simulink model "nms_3Dmodel_nonlin"  (R2019a)
settings: Solver=ode15s  StartTime=0.0  StopTime=10  FixedStep=1e-3  RelTol=1e-3  AbsTol=1e-4  EnableMultiTasking=on
InitFcn:
  | runScripts;
undefined symbols (not defined in the file or in its folder): ankle_height, c, c_jointstop, CtrlPar_FP, CtrlPar_FP_R, CtrlPar_LL, CtrlPar_St, CtrlPar_St_R, CtrlPar_Sw, CtrlPar_Sw_R, CtrlPar_theta0, CtrlPar_Tr, CtrlPar_Tr_R, D12_F, D12_S, D12_T, D12z_T, D13_F, D1G_F, D1G_HAT, D1G_S, D1G_T, D1Gy_F, d_fBall, d_fHeel, DeltaThRef, dt, eref, FmaxBFSH, FmaxGAS, FmaxGLU, FmaxHAB, FmaxHAD, FmaxHAM, FmaxHFL, FmaxRF, FmaxSOL, FmaxTA, FmaxVAS, In_F, In_HAT, In_S, In_T, init_a_tgt, init_a_tgtR, Inx_F, Inx_HAT, Inx_S, Inx_T, Iny_F, Iny_HAT, Iny_S, Iny_T, K, k_gn, k_gt, k_pressure, leg_l, LongDelay, LongLoopDelay ... (+139)
libraries: mblibv1 x89, simulink x44, simulink_extras x38
(part 11 of 13)

== system nms_3Dmodel_nonlin/Muscle Actuation Layer/R RF/PE force-length relation ==
  note: Parallel Elasticity PE
  lce [lopt] : Inport
  Constant3 : Constant
  Math Function2 : Math  Operator=square  SaturateOnIntegerOverflow=on
  Mux : Mux  Inputs=2
  Sum1 : Sum  Inputs=|+-  SaturateOnIntegerOverflow=on  InputSameDT=on  OutDataTypeStr=Inherit: Same as first input
  force above slack length : Fcn  Expr=u(2) * (u(1)>1)
  reference strain [lopt] : Constant  Value=w
  relative strain : Product  Inputs=*/
  fpe [Fmax] : Outport
  wires:
  Mux/1 -> force above slack length/1
  lce [lopt]/1 -> Mux/1, Sum1/1
  Constant3/1 -> Sum1/2
  Sum1/1 -> relative strain/1
  reference strain [lopt]/1 -> relative strain/2
  relative strain/1 -> Math Function2/1
  Math Function2/1 -> Mux/2
  force above slack length/1 -> fpe [Fmax]/1

== system nms_3Dmodel_nonlin/Muscle Actuation Layer/R RF/SE force-length relation ==
  note: SE Force-Length Relationship
  lse [lslack] : Inport
  Constant1 : Constant
  Math Function : Math  Operator=square  SaturateOnIntegerOverflow=on
  Mux : Mux  Inputs=2
  Sum4 : Sum  Inputs=|+-  SaturateOnIntegerOverflow=on  InputSameDT=on  OutDataTypeStr=Inherit: Same as first input
  force above slack length : Fcn  Expr=u(2)*(u(1)>1)
  reference strain [lslack] : Constant  Value=eref
  relative strain : Product  Inputs=*/
  fse [Fmax] : Outport
  wires:
  Mux/1 -> force above slack length/1
  force above slack length/1 -> fse [Fmax]/1
  Math Function/1 -> Mux/2
  lse [lslack]/1 -> Mux/1, Sum4/1
  relative strain/1 -> Math Function/1
  reference strain [lslack]/1 -> relative strain/2
  Sum4/1 -> relative strain/1
  Constant1/1 -> Sum4/2

== system nms_3Dmodel_nonlin/Muscle Actuation Layer/R SOL/BE force-length relation ==
  note: Buffer Elasticity BE
  lce [lopt] : Inport
  Constant1 : Constant  Value=1-w
  Math Function : Math  Operator=square  SaturateOnIntegerOverflow=on
  Mux1 : Mux  Inputs=2
  Sum4 : Sum  Inputs=|+-  SaturateOnIntegerOverflow=on  InputSameDT=on  OutDataTypeStr=Inherit: Same as first input
  force above slack length : Fcn  Expr=u(2)*(u(1)<0)
  reference strain [lslack] : Constant  Value=w/2
  relative strain : Product  Inputs=*/
  fbe [Fmax] : Outport
  wires:
  lce [lopt]/1 -> Sum4/1
  Mux1/1 -> force above slack length/1
  force above slack length/1 -> fbe [Fmax]/1
  Math Function/1 -> Mux1/2
  relative strain/1 -> Math Function/1
  reference strain [lslack]/1 -> relative strain/2
  Sum4/1 -> relative strain/1, Mux1/1
  Constant1/1 -> Sum4/2

== system nms_3Dmodel_nonlin/Muscle Actuation Layer/R SOL/CE force-length relation ==
  note: CE Force-Length Relationship
  lce [lopt] : Inport
  Abs : Abs
  Constant1 : Constant
  Constant2 : Constant  Value=3
  Gain : Gain  Gain=log(c)
  Math Function : Math  SaturateOnIntegerOverflow=on
  Math Function1 : Math  Operator=pow  SaturateOnIntegerOverflow=on
  Sum4 : Sum  Inputs=|+-  SaturateOnIntegerOverflow=on  InputSameDT=on  OutDataTypeStr=Inherit: Same as first input
  normalized position : Product  Inputs=*/
  relative width : Constant  Value=w
  fce [Fmax] : Outport
  wires:
  lce [lopt]/1 -> Sum4/1
  relative width/1 -> normalized position/2
  Constant1/1 -> Sum4/2
  Sum4/1 -> Abs/1
  Abs/1 -> normalized position/1
  normalized position/1 -> Math Function1/1
  Constant2/1 -> Math Function1/2
  Math Function1/1 -> Gain/1
  Gain/1 -> Math Function/1
  Math Function/1 -> fce [Fmax]/1

== system nms_3Dmodel_nonlin/Muscle Actuation Layer/R SOL/CE inverse force-velocity relation ==
  note: CE Inverse Force-Velocity Relationship
  Fv[Fmax] : Inport
  1 : Product  Inputs=/*
  Constant{1,3..4,8} (4 alike) : Constant
  Constant2 : Constant  Value=N
  Constant5 : Constant  Value=N
  Curvature : Gain  Gain=K  SaturateOnIntegerOverflow=on  OutDataTypeStr=Inherit: Same as input  ParamDataTypeStr=Inherit: Same as input
  Curvature1 : Gain  Gain=7.56*K  SaturateOnIntegerOverflow=on  OutDataTypeStr=Inherit: Same as input  ParamDataTypeStr=Inherit: Same as input
  Mux : Mux  Inputs=2
  Mux1 : Mux  Inputs=3
  Mux2 : Mux  Inputs=3
  Slope : Gain  Gain=1e-2  SaturateOnIntegerOverflow=on  OutDataTypeStr=Inherit: Same as input  ParamDataTypeStr=Inherit: Same as input
  Sum1 : Sum  Inputs=|++  SaturateOnIntegerOverflow=on  InputSameDT=on  OutDataTypeStr=Inherit: Same as first input
  Sum2 : Sum  SaturateOnIntegerOverflow=on  InputSameDT=on  OutDataTypeStr=Inherit: Same as first input
  Sum3 : Sum  Inputs=++|  SaturateOnIntegerOverflow=on  InputSameDT=on  OutDataTypeStr=Inherit: Same as first input
  Sum4 : Sum  Inputs=|+-  SaturateOnIntegerOverflow=on  InputSameDT=on  OutDataTypeStr=Inherit: Same as first input
  Sum5 : Sum  Inputs=|-+  SaturateOnIntegerOverflow=on  InputSameDT=on  OutDataTypeStr=Inherit: Same as first input
  Sum6 : Sum  Inputs=-+|  SaturateOnIntegerOverflow=on  InputSameDT=on  OutDataTypeStr=Inherit: Same as first input
  Sum7 : Sum  Inputs=|++  SaturateOnIntegerOverflow=on  InputSameDT=on  OutDataTypeStr=Inherit: Same as first input
  Sum8 : Sum  Inputs=+-|  SaturateOnIntegerOverflow=on  InputSameDT=on  OutDataTypeStr=Inherit: Same as first input
  Sum9 : Sum  SaturateOnIntegerOverflow=on  InputSameDT=on  OutDataTypeStr=Inherit: Same as first input
  concentric branch : Fcn  Expr=u(1) * (u(2)<=1)
  excentric branch : Fcn  Expr=u(2) * (u(1)>1)*(u(1)<=u(3))
  excentric overshoot : Fcn  Expr=u(3) * (u(2)>u(1))
  v_concentric : Product  Inputs=*/
  v_excentric <N : Product  Inputs=*/
  v[vmax] : Outport
  wires:
  Curvature/1 -> Sum3/2
  Constant1/1 -> Sum4/2, Sum3/1
  Sum4/1 -> v_concentric/1
  Sum3/1 -> v_concentric/2
  1/1 -> Sum7/1, Curvature1/1
  Constant4/1 -> Sum7/2, Sum8/1
  Curvature1/1 -> Sum8/2
  Sum8/1 -> v_excentric <N/2
  Sum7/1 -> v_excentric <N/1
  v_concentric/1 -> Mux/1
  Fv[Fmax]/1 -> Sum4/1, Curvature/1, Sum6/2, Mux/2, Mux1/1, Mux2/2
  Sum9/1 -> v[vmax]/1
  Sum2/1 -> Sum9/2
  excentric overshoot/1 -> Sum2/2
  Slope/1 -> Sum1/1
  Constant8/1 -> Sum1/2
  Sum6/1 -> 1/2, Slope/1
  Constant2/1 -> Sum6/1, Sum5/2
  Sum5/1 -> 1/1
  Constant3/1 -> Sum5/1
  Mux/1 -> concentric branch/1
  Mux1/1 -> excentric branch/1
  v_excentric <N/1 -> Mux1/2
  Mux2/1 -> excentric overshoot/1
  concentric branch/1 -> Sum9/1
  excentric branch/1 -> Sum2/1
  Constant5/1 -> Mux1/3, Mux2/1
  Sum1/1 -> Mux2/3

== system nms_3Dmodel_nonlin/Muscle Actuation Layer/R SOL/PE force-length relation ==
  note: Parallel Elasticity PE
  lce [lopt] : Inport
  Constant3 : Constant
  Math Function2 : Math  Operator=square  SaturateOnIntegerOverflow=on
  Mux : Mux  Inputs=2
  Sum1 : Sum  Inputs=|+-  SaturateOnIntegerOverflow=on  InputSameDT=on  OutDataTypeStr=Inherit: Same as first input
  force above slack length : Fcn  Expr=u(2) * (u(1)>1)
  reference strain [lopt] : Constant  Value=w
  relative strain : Product  Inputs=*/
  fpe [Fmax] : Outport
  wires:
  Mux/1 -> force above slack length/1
  lce [lopt]/1 -> Mux/1, Sum1/1
  Constant3/1 -> Sum1/2
  Sum1/1 -> relative strain/1
  reference strain [lopt]/1 -> relative strain/2
  relative strain/1 -> Math Function2/1
  Math Function2/1 -> Mux/2
  force above slack length/1 -> fpe [Fmax]/1

== system nms_3Dmodel_nonlin/Muscle Actuation Layer/R SOL/SE force-length relation ==
  note: SE Force-Length Relationship
  lse [lslack] : Inport
  Constant1 : Constant
  Math Function : Math  Operator=square  SaturateOnIntegerOverflow=on
  Mux : Mux  Inputs=2
  Sum4 : Sum  Inputs=|+-  SaturateOnIntegerOverflow=on  InputSameDT=on  OutDataTypeStr=Inherit: Same as first input
  force above slack length : Fcn  Expr=u(2)*(u(1)>1)
  reference strain [lslack] : Constant  Value=eref
  relative strain : Product  Inputs=*/
  fse [Fmax] : Outport
  wires:
  Mux/1 -> force above slack length/1
  force above slack length/1 -> fse [Fmax]/1
  Math Function/1 -> Mux/2
  lse [lslack]/1 -> Mux/1, Sum4/1
  relative strain/1 -> Math Function/1
  reference strain [lslack]/1 -> relative strain/2
  Sum4/1 -> relative strain/1
  Constant1/1 -> Sum4/2

== system nms_3Dmodel_nonlin/Muscle Actuation Layer/R TA/BE force-length relation ==
  note: Buffer Elasticity BE
  lce [lopt] : Inport
  Constant1 : Constant  Value=1-w
  Math Function : Math  Operator=square  SaturateOnIntegerOverflow=on
  Mux1 : Mux  Inputs=2
  Sum4 : Sum  Inputs=|+-  SaturateOnIntegerOverflow=on  InputSameDT=on  OutDataTypeStr=Inherit: Same as first input
  force above slack length : Fcn  Expr=u(2)*(u(1)<0)
  reference strain [lslack] : Constant  Value=w/2
  relative strain : Product  Inputs=*/
  fbe [Fmax] : Outport
  wires:
  lce [lopt]/1 -> Sum4/1
  Mux1/1 -> force above slack length/1
  force above slack length/1 -> fbe [Fmax]/1
  Math Function/1 -> Mux1/2
  relative strain/1 -> Math Function/1
  reference strain [lslack]/1 -> relative strain/2
  Sum4/1 -> relative strain/1, Mux1/1
  Constant1/1 -> Sum4/2

== system nms_3Dmodel_nonlin/Muscle Actuation Layer/R TA/CE force-length relation ==
  note: CE Force-Length Relationship
  lce [lopt] : Inport
  Abs : Abs
  Constant1 : Constant
  Constant2 : Constant  Value=3
  Gain : Gain  Gain=log(c)
  Math Function : Math  SaturateOnIntegerOverflow=on
  Math Function1 : Math  Operator=pow  SaturateOnIntegerOverflow=on
  Sum4 : Sum  Inputs=|+-  SaturateOnIntegerOverflow=on  InputSameDT=on  OutDataTypeStr=Inherit: Same as first input
  normalized position : Product  Inputs=*/
  relative width : Constant  Value=w
  fce [Fmax] : Outport
  wires:
  Math Function/1 -> fce [Fmax]/1
  Gain/1 -> Math Function/1
  Math Function1/1 -> Gain/1
  Constant2/1 -> Math Function1/2
  normalized position/1 -> Math Function1/1
  Abs/1 -> normalized position/1
  Sum4/1 -> Abs/1
  Constant1/1 -> Sum4/2
  relative width/1 -> normalized position/2
  lce [lopt]/1 -> Sum4/1

== system nms_3Dmodel_nonlin/Muscle Actuation Layer/R TA/CE inverse force-velocity relation ==
  note: CE Inverse Force-Velocity Relationship
  Fv[Fmax] : Inport
  1 : Product  Inputs=/*
  Constant{1,3..4,8} (4 alike) : Constant
  Constant2 : Constant  Value=N
  Constant5 : Constant  Value=N
  Curvature : Gain  Gain=K  SaturateOnIntegerOverflow=on  OutDataTypeStr=Inherit: Same as input  ParamDataTypeStr=Inherit: Same as input
  Curvature1 : Gain  Gain=7.56*K  SaturateOnIntegerOverflow=on  OutDataTypeStr=Inherit: Same as input  ParamDataTypeStr=Inherit: Same as input
  Mux : Mux  Inputs=2
  Mux1 : Mux  Inputs=3
  Mux2 : Mux  Inputs=3
  Slope : Gain  Gain=1e-2  SaturateOnIntegerOverflow=on  OutDataTypeStr=Inherit: Same as input  ParamDataTypeStr=Inherit: Same as input
  Sum1 : Sum  Inputs=|++  SaturateOnIntegerOverflow=on  InputSameDT=on  OutDataTypeStr=Inherit: Same as first input
  Sum2 : Sum  SaturateOnIntegerOverflow=on  InputSameDT=on  OutDataTypeStr=Inherit: Same as first input
  Sum3 : Sum  Inputs=++|  SaturateOnIntegerOverflow=on  InputSameDT=on  OutDataTypeStr=Inherit: Same as first input
  Sum4 : Sum  Inputs=|+-  SaturateOnIntegerOverflow=on  InputSameDT=on  OutDataTypeStr=Inherit: Same as first input
  Sum5 : Sum  Inputs=|-+  SaturateOnIntegerOverflow=on  InputSameDT=on  OutDataTypeStr=Inherit: Same as first input
  Sum6 : Sum  Inputs=-+|  SaturateOnIntegerOverflow=on  InputSameDT=on  OutDataTypeStr=Inherit: Same as first input
  Sum7 : Sum  Inputs=|++  SaturateOnIntegerOverflow=on  InputSameDT=on  OutDataTypeStr=Inherit: Same as first input
  Sum8 : Sum  Inputs=+-|  SaturateOnIntegerOverflow=on  InputSameDT=on  OutDataTypeStr=Inherit: Same as first input
  Sum9 : Sum  SaturateOnIntegerOverflow=on  InputSameDT=on  OutDataTypeStr=Inherit: Same as first input
  concentric branch : Fcn  Expr=u(1) * (u(2)<=1)
  excentric branch : Fcn  Expr=u(2) * (u(1)>1)*(u(1)<=u(3))
  excentric overshoot : Fcn  Expr=u(3) * (u(2)>u(1))
  v_concentric : Product  Inputs=*/
  v_excentric <N : Product  Inputs=*/
  v[vmax] : Outport
  wires:
  Sum1/1 -> Mux2/3
  Constant5/1 -> Mux2/1, Mux1/3
  excentric branch/1 -> Sum2/1
  concentric branch/1 -> Sum9/1
  Mux2/1 -> excentric overshoot/1
  v_excentric <N/1 -> Mux1/2
  Mux1/1 -> excentric branch/1
  Mux/1 -> concentric branch/1
  Constant3/1 -> Sum5/1
  Sum5/1 -> 1/1
  Constant2/1 -> Sum5/2, Sum6/1
  Sum6/1 -> Slope/1, 1/2
  Constant8/1 -> Sum1/2
  Slope/1 -> Sum1/1
  excentric overshoot/1 -> Sum2/2
  Sum2/1 -> Sum9/2
  Sum9/1 -> v[vmax]/1
  Fv[Fmax]/1 -> Mux2/2, Mux1/1, Mux/2, Sum6/2, Curvature/1, Sum4/1
  v_concentric/1 -> Mux/1
  Sum7/1 -> v_excentric <N/1
  Sum8/1 -> v_excentric <N/2
  Curvature1/1 -> Sum8/2
  Constant4/1 -> Sum8/1, Sum7/2
  1/1 -> Curvature1/1, Sum7/1
  Sum3/1 -> v_concentric/2
  Sum4/1 -> v_concentric/1
  Constant1/1 -> Sum3/1, Sum4/2
  Curvature/1 -> Sum3/2

== system nms_3Dmodel_nonlin/Muscle Actuation Layer/R TA/PE force-length relation ==
  note: Parallel Elasticity PE
  lce [lopt] : Inport
  Constant3 : Constant
  Math Function2 : Math  Operator=square  SaturateOnIntegerOverflow=on
  Mux : Mux  Inputs=2
  Sum1 : Sum  Inputs=|+-  SaturateOnIntegerOverflow=on  InputSameDT=on  OutDataTypeStr=Inherit: Same as first input
  force above slack length : Fcn  Expr=u(2) * (u(1)>1)
  reference strain [lopt] : Constant  Value=w
  relative strain : Product  Inputs=*/
  fpe [Fmax] : Outport
  wires:
  Mux/1 -> force above slack length/1
  lce [lopt]/1 -> Mux/1, Sum1/1
  Constant3/1 -> Sum1/2
  Sum1/1 -> relative strain/1
  reference strain [lopt]/1 -> relative strain/2
  relative strain/1 -> Math Function2/1
  Math Function2/1 -> Mux/2
  force above slack length/1 -> fpe [Fmax]/1

== system nms_3Dmodel_nonlin/Muscle Actuation Layer/R TA/SE force-length relation ==
  note: SE Force-Length Relationship
  lse [lslack] : Inport
  Constant1 : Constant
  Math Function : Math  Operator=square  SaturateOnIntegerOverflow=on
  Mux : Mux  Inputs=2
  Sum4 : Sum  Inputs=|+-  SaturateOnIntegerOverflow=on  InputSameDT=on  OutDataTypeStr=Inherit: Same as first input
  force above slack length : Fcn  Expr=u(2)*(u(1)>1)
  reference strain [lslack] : Constant  Value=eref
  relative strain : Product  Inputs=*/
  fse [Fmax] : Outport
  wires:
  Mux/1 -> force above slack length/1
  force above slack length/1 -> fse [Fmax]/1
  Math Function/1 -> Mux/2
  lse [lslack]/1 -> Mux/1, Sum4/1
  relative strain/1 -> Math Function/1
  reference strain [lslack]/1 -> relative strain/2
  Sum4/1 -> relative strain/1
  Constant1/1 -> Sum4/2

== system nms_3Dmodel_nonlin/Muscle Actuation Layer/R VAS/BE force-length relation ==
  note: Buffer Elasticity BE
  lce [lopt] : Inport
  Constant1 : Constant  Value=1-w
  Math Function : Math  Operator=square  SaturateOnIntegerOverflow=on
  Mux1 : Mux  Inputs=2
  Sum4 : Sum  Inputs=|+-  SaturateOnIntegerOverflow=on  InputSameDT=on  OutDataTypeStr=Inherit: Same as first input
  force above slack length : Fcn  Expr=u(2)*(u(1)<0)
  reference strain [lslack] : Constant  Value=w/2
  relative strain : Product  Inputs=*/
  fbe [Fmax] : Outport
  wires:
  lce [lopt]/1 -> Sum4/1
  Mux1/1 -> force above slack length/1
  force above slack length/1 -> fbe [Fmax]/1
  Math Function/1 -> Mux1/2
  relative strain/1 -> Math Function/1
  reference strain [lslack]/1 -> relative strain/2
  Sum4/1 -> relative strain/1, Mux1/1
  Constant1/1 -> Sum4/2

== system nms_3Dmodel_nonlin/Muscle Actuation Layer/R VAS/CE force-length relation ==
  note: CE Force-Length Relationship
  lce [lopt] : Inport
  Abs : Abs
  Constant1 : Constant
  Constant2 : Constant  Value=3
  Gain : Gain  Gain=log(c)
  Math Function : Math  SaturateOnIntegerOverflow=on
  Math Function1 : Math  Operator=pow  SaturateOnIntegerOverflow=on
  Sum4 : Sum  Inputs=|+-  SaturateOnIntegerOverflow=on  InputSameDT=on  OutDataTypeStr=Inherit: Same as first input
  normalized position : Product  Inputs=*/
  relative width : Constant  Value=w
  fce [Fmax] : Outport
  wires:
  lce [lopt]/1 -> Sum4/1
  relative width/1 -> normalized position/2
  Constant1/1 -> Sum4/2
  Sum4/1 -> Abs/1
  Abs/1 -> normalized position/1
  normalized position/1 -> Math Function1/1
  Constant2/1 -> Math Function1/2
  Math Function1/1 -> Gain/1
  Gain/1 -> Math Function/1
  Math Function/1 -> fce [Fmax]/1

== system nms_3Dmodel_nonlin/Muscle Actuation Layer/R VAS/CE inverse force-velocity relation ==
  note: CE Inverse Force-Velocity Relationship
  Fv[Fmax] : Inport
  1 : Product  Inputs=/*
  Constant{1,3..4,8} (4 alike) : Constant
  Constant2 : Constant  Value=N
  Constant5 : Constant  Value=N
  Curvature : Gain  Gain=K  SaturateOnIntegerOverflow=on  OutDataTypeStr=Inherit: Same as input  ParamDataTypeStr=Inherit: Same as input
  Curvature1 : Gain  Gain=7.56*K  SaturateOnIntegerOverflow=on  OutDataTypeStr=Inherit: Same as input  ParamDataTypeStr=Inherit: Same as input
  Mux : Mux  Inputs=2
  Mux1 : Mux  Inputs=3
  Mux2 : Mux  Inputs=3
  Slope : Gain  Gain=1e-2  SaturateOnIntegerOverflow=on  OutDataTypeStr=Inherit: Same as input  ParamDataTypeStr=Inherit: Same as input
  Sum1 : Sum  Inputs=|++  SaturateOnIntegerOverflow=on  InputSameDT=on  OutDataTypeStr=Inherit: Same as first input
  Sum2 : Sum  SaturateOnIntegerOverflow=on  InputSameDT=on  OutDataTypeStr=Inherit: Same as first input
  Sum3 : Sum  Inputs=++|  SaturateOnIntegerOverflow=on  InputSameDT=on  OutDataTypeStr=Inherit: Same as first input
  Sum4 : Sum  Inputs=|+-  SaturateOnIntegerOverflow=on  InputSameDT=on  OutDataTypeStr=Inherit: Same as first input
  Sum5 : Sum  Inputs=|-+  SaturateOnIntegerOverflow=on  InputSameDT=on  OutDataTypeStr=Inherit: Same as first input
  Sum6 : Sum  Inputs=-+|  SaturateOnIntegerOverflow=on  InputSameDT=on  OutDataTypeStr=Inherit: Same as first input
  Sum7 : Sum  Inputs=|++  SaturateOnIntegerOverflow=on  InputSameDT=on  OutDataTypeStr=Inherit: Same as first input
  Sum8 : Sum  Inputs=+-|  SaturateOnIntegerOverflow=on  InputSameDT=on  OutDataTypeStr=Inherit: Same as first input
  Sum9 : Sum  SaturateOnIntegerOverflow=on  InputSameDT=on  OutDataTypeStr=Inherit: Same as first input
  concentric branch : Fcn  Expr=u(1) * (u(2)<=1)
  excentric branch : Fcn  Expr=u(2) * (u(1)>1)*(u(1)<=u(3))
  excentric overshoot : Fcn  Expr=u(3) * (u(2)>u(1))
  v_concentric : Product  Inputs=*/
  v_excentric <N : Product  Inputs=*/
  v[vmax] : Outport
  wires:
  Curvature/1 -> Sum3/2
  Constant1/1 -> Sum4/2, Sum3/1
  Sum4/1 -> v_concentric/1
  Sum3/1 -> v_concentric/2
  1/1 -> Sum7/1, Curvature1/1
  Constant4/1 -> Sum7/2, Sum8/1
  Curvature1/1 -> Sum8/2
  Sum8/1 -> v_excentric <N/2
  Sum7/1 -> v_excentric <N/1
  v_concentric/1 -> Mux/1
  Fv[Fmax]/1 -> Sum4/1, Curvature/1, Sum6/2, Mux/2, Mux1/1, Mux2/2
  Sum9/1 -> v[vmax]/1
  Sum2/1 -> Sum9/2
  excentric overshoot/1 -> Sum2/2
  Slope/1 -> Sum1/1
  Constant8/1 -> Sum1/2
  Sum6/1 -> 1/2, Slope/1
  Constant2/1 -> Sum6/1, Sum5/2
  Sum5/1 -> 1/1
  Constant3/1 -> Sum5/1
  Mux/1 -> concentric branch/1
  Mux1/1 -> excentric branch/1
  v_excentric <N/1 -> Mux1/2
  Mux2/1 -> excentric overshoot/1
  concentric branch/1 -> Sum9/1
  excentric branch/1 -> Sum2/1
  Constant5/1 -> Mux1/3, Mux2/1
  Sum1/1 -> Mux2/3

== system nms_3Dmodel_nonlin/Muscle Actuation Layer/R VAS/PE force-length relation ==
  note: Parallel Elasticity PE
  lce [lopt] : Inport
  Constant3 : Constant
  Math Function2 : Math  Operator=square  SaturateOnIntegerOverflow=on
  Mux : Mux  Inputs=2
  Sum1 : Sum  Inputs=|+-  SaturateOnIntegerOverflow=on  InputSameDT=on  OutDataTypeStr=Inherit: Same as first input
  force above slack length : Fcn  Expr=u(2) * (u(1)>1)
  reference strain [lopt] : Constant  Value=w
  relative strain : Product  Inputs=*/
  fpe [Fmax] : Outport
  wires:
  Mux/1 -> force above slack length/1
  lce [lopt]/1 -> Mux/1, Sum1/1
  Constant3/1 -> Sum1/2
  Sum1/1 -> relative strain/1
  reference strain [lopt]/1 -> relative strain/2
  relative strain/1 -> Math Function2/1
  Math Function2/1 -> Mux/2
  force above slack length/1 -> fpe [Fmax]/1

== system nms_3Dmodel_nonlin/Muscle Actuation Layer/R VAS/SE force-length relation ==
  note: SE Force-Length Relationship
  lse [lslack] : Inport
  Constant1 : Constant
  Math Function : Math  Operator=square  SaturateOnIntegerOverflow=on
  Mux : Mux  Inputs=2
  Sum4 : Sum  Inputs=|+-  SaturateOnIntegerOverflow=on  InputSameDT=on  OutDataTypeStr=Inherit: Same as first input
  force above slack length : Fcn  Expr=u(2)*(u(1)>1)
  reference strain [lslack] : Constant  Value=eref
  relative strain : Product  Inputs=*/
  fse [Fmax] : Outport
  wires:
  Mux/1 -> force above slack length/1
  force above slack length/1 -> fse [Fmax]/1
  Math Function/1 -> Mux/2
  lse [lslack]/1 -> Mux/1, Sum4/1
  relative strain/1 -> Math Function/1
  reference strain [lslack]/1 -> relative strain/2
  Sum4/1 -> relative strain/1
  Constant1/1 -> Sum4/2

== system nms_3Dmodel_nonlin/Neural Control Layer (Spinal Cord Control)/L Swing Phase (sagittal)/kneei_flexion from alpha ==
  note: Knee Phase i
  SBFSH : Inport
  Enable : EnablePort  StatesWhenEnabling=reset  ZeroCross=off
  SBFSH_Sw_ki : Outport  OutputWhenDisabled=reset  InitialOutput=0
  wires:
  SBFSH/1 -> SBFSH_Sw_ki/1

== system nms_3Dmodel_nonlin/Neural Control Layer (Spinal Cord Control)/L Swing Phase (sagittal)/kneeii_damp and hold &kneeiii_leg stop &kneeiv_stance preparation ==
  note: Knee Phase i
  CtrlPar : Inport
  a_tgt : Inport  Port=2
  LceRF : Inport  Port=3
  LceHAM : Inport  Port=4
  VceHAM : Inport  Port=5
  VceVAS : Inport  Port=6
  VceBFSH : Inport  Port=7
  VceRF : Inport  Port=8
  LceHFL : Inport  Port=9
  LceGLU : Inport  Port=10
  LceVAS : Inport  Port=11
  Enable : EnablePort  StatesWhenEnabling=reset  ZeroCross=off
  Compare To Constant : simulink/Logic and Bit Operations/Compare To Constant  relop=<=  const=0  OutDataTypeStr=uint8  ZeroCross=off
  Constant1 : Constant  Value=0  OutDataTypeStr=boolean
  Constant2 : Constant  Value=0  OutDataTypeStr=boolean
  Constant3 : Constant  Value=0  OutDataTypeStr=boolean
  Constant4 : Constant
  Constant5 : Constant
  Demux1 : Demux  Outputs=5
  Divide1 : Product
  Divide2 : Product
  Logical Operator : Logic  Operator=NOT  AllPortsSameDT=off  OutDataTypeStr=boolean
  Logical Operator1 : Logic  AllPortsSameDT=off  OutDataTypeStr=boolean
  Relational Operator : RelationalOperator  Operator=<=  OutDataTypeStr=boolean  ZeroCross=off  RndMeth=Nearest
  Relational Operator1 : RelationalOperator  OutDataTypeStr=boolean  ZeroCross=off  RndMeth=Nearest
  S-R Flip-Flop : simulink_extras/Flip Flops/S-R Flip-Flop  initial_condition=0
  S-R Flip-Flop1 : simulink_extras/Flip Flops/S-R Flip-Flop  initial_condition=0
  S-R Flip-Flop2 : simulink_extras/Flip Flops/S-R Flip-Flop  initial_condition=0
  Sum1 : Sum  Inputs=+-|  SaturateOnIntegerOverflow=on  InputSameDT=on  OutDataTypeStr=Inherit: Same as first input
  Sum2 : Sum  Inputs=++|  SaturateOnIntegerOverflow=on  InputSameDT=on  OutDataTypeStr=Inherit: Same as first input
  Sum3 : Sum  Inputs=+-|  SaturateOnIntegerOverflow=on  InputSameDT=on  OutDataTypeStr=Inherit: Same as first input
  Sum4 : Sum  Inputs=+-|  SaturateOnIntegerOverflow=on  InputSameDT=on  OutDataTypeStr=Inherit: Same as first input
  Sum5 : Sum  Inputs=++|  SaturateOnIntegerOverflow=on  InputSameDT=on  OutDataTypeStr=Inherit: Same as first input
  Terminator : Terminator
  Terminator1 : Terminator
  Terminator2 : Terminator
  kneeii_damp and hold : Subsystem  TreatAsAtomicUnit=on
  kneeiii_leg stop : Subsystem  TreatAsAtomicUnit=on
  kneeiv_stance preparation : Subsystem  TreatAsAtomicUnit=on
  parSwKii : Selector  InputPortWidth=Sw_i  IndexOptions=Index vector (dialog)  Indices=parSwKii_i  OutputSizes=1
  parSwKiii : Selector  InputPortWidth=Sw_i  IndexOptions=Index vector (dialog)  Indices=parSwKiii_i  OutputSizes=1
  parSwKiv : Selector  InputPortWidth=Sw_i  IndexOptions=Index vector (dialog)  Indices=parSwKiv_i  OutputSizes=1
  parSwPhii : Selector  InputPortWidth=Sw_i  IndexOptions=Index vector (dialog)  Indices=parSwPhii_i  OutputSizes=1
  SRF_Sw_kii : Outport  OutputWhenDisabled=reset  InitialOutput=0
  SBFSH_Sw_kii : Outport  Port=2  OutputWhenDisabled=reset  InitialOutput=0
  SHAM_Sw_kiii : Outport  Port=3  OutputWhenDisabled=reset  InitialOutput=0
  SBFSH_Sw_kiii : Outport  Port=4  OutputWhenDisabled=reset  InitialOutput=0
  SGAS_Sw_kiii : Outport  Port=5  OutputWhenDisabled=reset  InitialOutput=0
  SHFL_Sw_kiv : Outport  Port=6  OutputWhenDisabled=reset  InitialOutput=0
  SGLU_Sw_kiv : Outport  Port=7  OutputWhenDisabled=reset  InitialOutput=0
  SVAS_Sw_kiv : Outport  Port=8  OutputWhenDisabled=reset  InitialOutput=0
  wires:
  Constant1/1 -> S-R Flip-Flop/2
  S-R Flip-Flop/2 -> Terminator/1
  Relational Operator/1 -> S-R Flip-Flop/1
  Constant2/1 -> S-R Flip-Flop1/2
  S-R Flip-Flop1/2 -> Terminator1/1
  Relational Operator1/1 -> S-R Flip-Flop1/1
  Constant3/1 -> S-R Flip-Flop2/2
  S-R Flip-Flop2/2 -> Terminator2/1
  Logical Operator1/1 -> S-R Flip-Flop2/1
  CtrlPar/1 -> parSwKii/1, parSwKiii/1, parSwKiv/1, parSwPhii/1
  S-R Flip-Flop/1 -> Logical Operator/1
  parSwKii/1 -> kneeii_damp and hold/1(CtrlPar)
  S-R Flip-Flop1/1 -> kneeiii_leg stop/Enable, Logical Operator1/1
  S-R Flip-Flop2/1 -> kneeiv_stance preparation/Enable
  parSwKiii/1 -> kneeiii_leg stop/1(CtrlPar)
  parSwKiv/1 -> kneeiv_stance preparation/1(CtrlPar)
  kneeii_damp and hold/1(SRF_Sw_kii) -> SRF_Sw_kii/1
  kneeii_damp and hold/2(SBFSH_Sw_kii) -> SBFSH_Sw_kii/1
  kneeiii_leg stop/1(SHAM_Sw_kiii) -> SHAM_Sw_kiii/1
  kneeiii_leg stop/2(SKFL_Sw_kiii) -> SBFSH_Sw_kiii/1
  kneeiii_leg stop/3(SGAS_Sw_kiii) -> SGAS_Sw_kiii/1
  kneeiv_stance preparation/1(SHFL_Sw_kiv) -> SHFL_Sw_kiv/1
  kneeiv_stance preparation/2(SGLU_Sw_kiv) -> SGLU_Sw_kiv/1
  kneeiv_stance preparation/3(SVAS_Sw_kiv) -> SVAS_Sw_kiv/1
  parSwPhii/1 -> Demux1/1
  Demux1/1 -> Sum3/2  "aRef_RF"
  Sum3/1 -> Divide1/1
  Constant4/1 -> Sum5/1
  Divide1/1 -> Sum5/2
  a_tgt/1 -> Sum2/1, Sum3/1, kneeii_damp and hold/2(a_tgt), kneeiii_leg stop/2(a_tgt), kneeiv_stance preparation/2(a_tgt)
  Demux1/2 -> Divide1/2  "a2lopt_RF"
  Sum5/1 -> Relational Operator/2  "lceOffRF"
  LceRF/1 -> Relational Operator/1, kneeii_damp and hold/6(LceRF)
  Logical Operator/1 -> kneeii_damp and hold/Enable
  Demux1/3 -> Sum2/2  "a_del"
  Sum2/1 -> Sum1/1  "a_thr"
  Demux1/4 -> Sum1/2  "aRef_HAM"
  Sum1/1 -> Divide2/1
  Demux1/5 -> Divide2/2  "a2lopt_HAM"
  Constant5/1 -> Sum4/1
  Divide2/1 -> Sum4/2
  Sum4/1 -> Relational Operator1/2  "lceOffHAM"
  LceHAM/1 -> kneeiii_leg stop/3(LceHAM), Relational Operator1/1  "LceHAM"
  Compare To Constant/1 -> Logical Operator1/2
  VceHAM/1 -> Compare To Constant/1
  VceBFSH/1 -> kneeii_damp and hold/4(VceBFSH)
  VceRF/1 -> kneeii_damp and hold/5(VceRF)
  LceHFL/1 -> kneeiv_stance preparation/3(LceHFL)
  LceGLU/1 -> kneeiv_stance preparation/4(lceGLU)
  LceVAS/1 -> kneeiv_stance preparation/5(lceVAS)
  VceVAS/1 -> kneeii_damp and hold/3(VceVAS)

== system nms_3Dmodel_nonlin/Neural Control Layer (Spinal Cord Control)/R Swing Phase (sagittal)/kneei_flexion from alpha ==
  note: Knee Phase i
  SBFSH : Inport
  Enable : EnablePort  StatesWhenEnabling=reset  ZeroCross=off
  SBFSH_Sw_ki : Outport  OutputWhenDisabled=reset  InitialOutput=0
  wires:
  SBFSH/1 -> SBFSH_Sw_ki/1

== system nms_3Dmodel_nonlin/Neural Control Layer (Spinal Cord Control)/R Swing Phase (sagittal)/kneeii_damp and hold &kneeiii_leg stop &kneeiv_stance preparation ==
  note: Knee Phase i
  CtrlPar : Inport
  a_tgt : Inport  Port=2
  LceRF : Inport  Port=3
  LceHAM : Inport  Port=4
  VceHAM : Inport  Port=5
  VceVAS : Inport  Port=6
  VceBFSH : Inport  Port=7
  VceRF : Inport  Port=8
  LceHFL : Inport  Port=9
  LceGLU : Inport  Port=10
  LceVAS : Inport  Port=11
  Enable : EnablePort  StatesWhenEnabling=reset  ZeroCross=off
  Compare To Constant : simulink/Logic and Bit Operations/Compare To Constant  relop=<=  const=0  OutDataTypeStr=uint8  ZeroCross=off
  Constant1 : Constant  Value=0  OutDataTypeStr=boolean
  Constant2 : Constant  Value=0  OutDataTypeStr=boolean
  Constant3 : Constant  Value=0  OutDataTypeStr=boolean
  Constant4 : Constant
  Constant5 : Constant
  Demux1 : Demux  Outputs=5
  Divide1 : Product
  Divide2 : Product
  Logical Operator : Logic  Operator=NOT  AllPortsSameDT=off  OutDataTypeStr=boolean
  Logical Operator1 : Logic  AllPortsSameDT=off  OutDataTypeStr=boolean
  Relational Operator : RelationalOperator  Operator=<=  OutDataTypeStr=boolean  ZeroCross=off  RndMeth=Nearest
  Relational Operator1 : RelationalOperator  OutDataTypeStr=boolean  ZeroCross=off  RndMeth=Nearest
  S-R Flip-Flop : simulink_extras/Flip Flops/S-R Flip-Flop  initial_condition=0
  S-R Flip-Flop1 : simulink_extras/Flip Flops/S-R Flip-Flop  initial_condition=0
  S-R Flip-Flop2 : simulink_extras/Flip Flops/S-R Flip-Flop  initial_condition=0
  Sum1 : Sum  Inputs=+-|  SaturateOnIntegerOverflow=on  InputSameDT=on  OutDataTypeStr=Inherit: Same as first input
  Sum2 : Sum  Inputs=++|  SaturateOnIntegerOverflow=on  InputSameDT=on  OutDataTypeStr=Inherit: Same as first input
  Sum3 : Sum  Inputs=+-|  SaturateOnIntegerOverflow=on  InputSameDT=on  OutDataTypeStr=Inherit: Same as first input
  Sum4 : Sum  Inputs=+-|  SaturateOnIntegerOverflow=on  InputSameDT=on  OutDataTypeStr=Inherit: Same as first input
  Sum5 : Sum  Inputs=++|  SaturateOnIntegerOverflow=on  InputSameDT=on  OutDataTypeStr=Inherit: Same as first input
  Terminator : Terminator
  Terminator1 : Terminator
  Terminator2 : Terminator
  kneeii_damp and hold : Subsystem  TreatAsAtomicUnit=on
  kneeiii_leg stop : Subsystem  TreatAsAtomicUnit=on
  kneeiv_stance preparation : Subsystem  TreatAsAtomicUnit=on
  parSwKii : Selector  InputPortWidth=Sw_i  IndexOptions=Index vector (dialog)  Indices=parSwKii_i  OutputSizes=1
  parSwKiii : Selector  InputPortWidth=Sw_i  IndexOptions=Index vector (dialog)  Indices=parSwKiii_i  OutputSizes=1
  parSwKiv : Selector  InputPortWidth=Sw_i  IndexOptions=Index vector (dialog)  Indices=parSwKiv_i  OutputSizes=1
  parSwPhii : Selector  InputPortWidth=Sw_i  IndexOptions=Index vector (dialog)  Indices=parSwPhii_i  OutputSizes=1
  SRF_Sw_kii : Outport  OutputWhenDisabled=reset  InitialOutput=0
  SBFSH_Sw_kii : Outport  Port=2  OutputWhenDisabled=reset  InitialOutput=0
  SHAM_Sw_kiii : Outport  Port=3  OutputWhenDisabled=reset  InitialOutput=0
  SBFSH_Sw_kiii : Outport  Port=4  OutputWhenDisabled=reset  InitialOutput=0
  SGAS_Sw_kiii : Outport  Port=5  OutputWhenDisabled=reset  InitialOutput=0
  SHFL_Sw_kiv : Outport  Port=6  OutputWhenDisabled=reset  InitialOutput=0
  SGLU_Sw_kiv : Outport  Port=7  OutputWhenDisabled=reset  InitialOutput=0
  SVAS_Sw_kiv : Outport  Port=8  OutputWhenDisabled=reset  InitialOutput=0
  wires:
  Constant1/1 -> S-R Flip-Flop/2
  S-R Flip-Flop/2 -> Terminator/1
  Relational Operator/1 -> S-R Flip-Flop/1
  Constant2/1 -> S-R Flip-Flop1/2
  S-R Flip-Flop1/2 -> Terminator1/1
  Relational Operator1/1 -> S-R Flip-Flop1/1
  Constant3/1 -> S-R Flip-Flop2/2
  S-R Flip-Flop2/2 -> Terminator2/1
  Logical Operator1/1 -> S-R Flip-Flop2/1
  CtrlPar/1 -> parSwKii/1, parSwKiii/1, parSwKiv/1, parSwPhii/1
  S-R Flip-Flop/1 -> Logical Operator/1
  parSwKii/1 -> kneeii_damp and hold/1(CtrlPar)
  S-R Flip-Flop1/1 -> kneeiii_leg stop/Enable, Logical Operator1/1
  S-R Flip-Flop2/1 -> kneeiv_stance preparation/Enable
  parSwKiii/1 -> kneeiii_leg stop/1(CtrlPar)
  parSwKiv/1 -> kneeiv_stance preparation/1(CtrlPar)
  kneeii_damp and hold/1(SRF_Sw_kii) -> SRF_Sw_kii/1
  kneeii_damp and hold/2(SBFSH_Sw_kii) -> SBFSH_Sw_kii/1
  kneeiii_leg stop/1(SHAM_Sw_kiii) -> SHAM_Sw_kiii/1
  kneeiii_leg stop/2(SKFL_Sw_kiii) -> SBFSH_Sw_kiii/1
  kneeiii_leg stop/3(SGAS_Sw_kiii) -> SGAS_Sw_kiii/1
  kneeiv_stance preparation/1(SHFL_Sw_kiv) -> SHFL_Sw_kiv/1
  kneeiv_stance preparation/2(SGLU_Sw_kiv) -> SGLU_Sw_kiv/1
  kneeiv_stance preparation/3(SVAS_Sw_kiv) -> SVAS_Sw_kiv/1
  parSwPhii/1 -> Demux1/1
  Demux1/1 -> Sum3/2  "aRef_RF"
  Sum3/1 -> Divide1/1
  Constant4/1 -> Sum5/1
  Divide1/1 -> Sum5/2
  a_tgt/1 -> Sum2/1, Sum3/1, kneeii_damp and hold/2(a_tgt), kneeiii_leg stop/2(a_tgt), kneeiv_stance preparation/2(a_tgt)
  Demux1/2 -> Divide1/2  "a2lopt_RF"
  Sum5/1 -> Relational Operator/2  "lceOffRF"
  LceRF/1 -> kneeii_damp and hold/6(LceRF), Relational Operator/1
  Logical Operator/1 -> kneeii_damp and hold/Enable
  Demux1/3 -> Sum2/2  "a_del"
  Sum2/1 -> Sum1/1  "a_thr"
  Demux1/4 -> Sum1/2  "aRef_HAM"
  Sum1/1 -> Divide2/1
  Demux1/5 -> Divide2/2  "a2lopt_HAM"
  Constant5/1 -> Sum4/1
  Divide2/1 -> Sum4/2
  Sum4/1 -> Relational Operator1/2  "lceOffHAM"
  LceHAM/1 -> kneeiii_leg stop/3(LceHAM), Relational Operator1/1  "LceHAM"
  Compare To Constant/1 -> Logical Operator1/2
  VceHAM/1 -> Compare To Constant/1
  VceBFSH/1 -> kneeii_damp and hold/4(VceBFSH)
  VceRF/1 -> kneeii_damp and hold/5(VceRF)
  LceHFL/1 -> kneeiv_stance preparation/3(LceHFL)
  LceGLU/1 -> kneeiv_stance preparation/4(lceGLU)
  LceVAS/1 -> kneeiv_stance preparation/5(lceVAS)
  VceVAS/1 -> kneeii_damp and hold/3(VceVAS)

== system nms_3Dmodel_nonlin/Body Mechanics Layer/LLBall Cnt/3D Contact/Friction Switch ==
  note: Static/Kinetic Friction Switch
  Slide! : Inport
  Stick! : Inport  Port=2
  Memory : Memory
  S-R Flip-Flop : simulink_extras/Flip Flops/S-R Flip-Flop  initial_condition=0
  Terminator : Terminator
  Stiction : Outport
  wires:
  S-R Flip-Flop/1 -> Memory/1
  S-R Flip-Flop/2 -> Terminator/1
  Stick!/1 -> S-R Flip-Flop/1
  Slide!/1 -> S-R Flip-Flop/2
  Memory/1 -> Stiction/1

== system nms_3Dmodel_nonlin/Body Mechanics Layer/LLBall Cnt/3D Contact/Kinetic Friction Model ==
  note: Kinetic Friction Model
  note: Footpoint Determiner
  note: Sliding Limit Detector
  note: Normal Ground Friction
  note: Tangential Ground Friction
  vel [m/s m/s m/s] : Inport
  pos [m m m] : Inport  Port=2
  RefPt [m m m] : Inport  Port=3
  nVec [m m m] : Inport  Port=4
  Enable : EnablePort  StatesWhenEnabling=reset  ZeroCross=off
  Constant : Constant  Value=vLimit
  Constant1 : Constant  Value=[0 0 0 1]'
  Demux : Demux  Outputs=[3 1]
  FixPt Relational Operator : RelationalOperator  Operator=>  OutDataTypeStr=boolean  ZeroCross=off  RndMeth=Nearest
  Gain3 : Gain  Gain=k_gn
  Gain4 : Gain  Gain=1/v_gn_max
  Memory : Memory
  Mux1 : Mux  Inputs=2
  Mux2 : Mux  Inputs=2
  Negative : simulink/Logic and Bit Operations/Compare To Zero  relop=<  OutDataTypeStr=boolean
  Normal Axis Ground Force : Fcn  Expr="u(1)  *  (1-u(2)) * (u(2)<1)"
  Product : Product  RndMeth=Zero
  Product1 : Product  RndMeth=Zero
  Sum : Sum  Inputs=|+-
  Switch : Switch  Criteria=u2 > Threshold  Threshold=0.9*vLimit
      settings: AttributesFormatString=>%<Threshold>?
  Vector Norm : Subsystem
  d_n : DotProduct  InputSameDT=on  OutDataTypeStr=Inherit: Inherit via internal rule
  qnVec : Sum  Inputs=-+
  reverse direction : Gain  Gain=-1
  sliding friction coefficient : Gain  Gain=mu_slide
  tVec : Product  Inputs=*/  RndMeth=Zero
  v_n : DotProduct  InputSameDT=on  OutDataTypeStr=Inherit: Inherit via internal rule
  v_nVec : Product  RndMeth=Zero
  v_tVec : Sum  Inputs=-+|
  RefPtFP [m m m] : Outport  InitialOutput=[0 0 0]
      settings: AttributesFormatString=initial = '%<InitialOutput>'\nwhen disabled = '%<OutputWhenDisabled>'
  posFP [m m m] : Outport  Port=2  InitialOutput=[0 0 0]
      settings: AttributesFormatString=initial = '%<InitialOutput>'\nwhen disabled = '%<OutputWhenDisabled>'
  nVec FP [m m m] : Outport  Port=3  InitialOutput=0
      settings: AttributesFormatString=initial = '%<InitialOutput>'\nwhen disabled = '%<OutputWhenDisabled>'
  Stiction! : Outport  Port=4  OutputWhenDisabled=reset  InitialOutput=0
      settings: AttributesFormatString=initial = '%<InitialOutput>'\nwhen disabled = '%<OutputWhenDisabled>'
  F_t Slide [N N N] : Outport  Port=5  OutputWhenDisabled=reset  InitialOutput=[0 0 0]
      settings: AttributesFormatString=initial = '%<InitialOutput>'\nwhen disabled = '%<OutputWhenDisabled>'
  F_n Slide [N N N] : Outport  Port=6  OutputWhenDisabled=reset  InitialOutput=[0 0 0]
      settings: AttributesFormatString=initial = '%<InitialOutput>'\nwhen disabled = '%<OutputWhenDisabled>'
  wires:
  Normal Axis Ground Force/1 -> sliding friction coefficient/1, Product1/2
  Product/1 -> F_t Slide [N N N]/1
  FixPt Relational Operator/1 -> Stiction!/1
  Memory/1 -> FixPt Relational Operator/2
  Negative/1 -> FixPt Relational Operator/1, Memory/1
  Vector Norm/1(norm) -> Sum/1, Switch/2, Mux2/2
  Sum/1 -> Negative/1
  Constant/1 -> Sum/2
  Mux1/1 -> Normal Axis Ground Force/1
  Gain3/1 -> Mux1/1
  Gain4/1 -> Mux1/2
  nVec [m m m]/1 -> v_n/1, v_nVec/2, d_n/2, Product1/1, nVec FP [m m m]/1
  d_n/1 -> Gain3/1
  vel [m/s m/s m/s]/1 -> v_n/2, v_tVec/2
  v_n/1 -> Gain4/1, v_nVec/1
  v_nVec/1 -> v_tVec/1
  v_tVec/1 -> Vector Norm/1(vec), Mux2/1
  sliding friction coefficient/1 -> Product/1
  reverse direction/1 -> Product/2
  Product1/1 -> F_n Slide [N N N]/1
  tVec/1 -> reverse direction/1
  Constant1/1 -> Switch/3
  Mux2/1 -> Switch/1
  Switch/1 -> Demux/1
  Demux/2 -> tVec/2
  Demux/1 -> tVec/1
  pos [m m m]/1 -> posFP [m m m]/1, qnVec/1
  qnVec/1 -> d_n/1
  RefPt [m m m]/1 -> qnVec/2, RefPtFP [m m m]/1

== system nms_3Dmodel_nonlin/Body Mechanics Layer/LLBall Cnt/3D Contact/Static Friction Model ==
  note: Stiction Limit Detector
  note: Static Friction Model
  note: Zero multiplication prevents
      | horizontal friction model from
      | oscillating between static and kinetic
      | friction when the vertical force is zero but
      | the ground level is not yet reached
      | in the upward motion
  note: (distance to
      | surface)
  note: Tangential Ground Reaction Force
  pos [m] : Inport
  vel [m/s m/s m/s] : Inport  Port=2
  RefPtFP [m m m] : Inport  Port=3
  posFP [m] : Inport  Port=4
  nVecFP [m m m] : Inport  Port=5
  Enable : EnablePort  StatesWhenEnabling=reset  ZeroCross=off
  Abs : Abs
  Check Vertical Friction : Product  RndMeth=Zero
  Constant : Constant
  Dpos_n : DotProduct  InputSameDT=on  OutDataTypeStr=Inherit: Inherit via internal rule
  Dpos_nVec : Product  RndMeth=Zero
  Dpos_tVec : Sum  Inputs=|+-
  FixPt Relational Operator : RelationalOperator  Operator=>  OutDataTypeStr=boolean  ZeroCross=off  RndMeth=Nearest
  Gain : Gain  Gain=-1
  Gain1 : Gain  Gain=k_gn
  Gain2 : Gain  Gain=1/v_gn_max
  Gain3 : Gain  Gain=k_gt
  Gain5 : Gain  Gain=1/v_gt_max
  Memory : Memory
  Mux2 : Mux  Inputs=2
  Normal Ground Reaction Force : Fcn  Expr="u(1)  *  (1-u(2)) * (u(2)<1)"
  Positive : simulink/Logic and Bit Operations/Compare To Zero  relop=>  OutDataTypeStr=boolean
  Positive1 : simulink/Logic and Bit Operations/Compare To Zero  relop=>  OutDataTypeStr=boolean
  Product1 : Product  RndMeth=Zero
  Sign : Signum  ZeroCross=off
  Sum : Sum  Inputs=-+
  Sum1 : Sum  Inputs=|+-
  Sum2 : Sum  Inputs=|+-
  Vector Norm : Subsystem
  d_n : DotProduct  InputSameDT=on  OutDataTypeStr=Inherit: Inherit via internal rule
  stiction limit force : Gain  Gain=mu_stick
  sum : Sum  Inputs=++|
  tVec1 : Product  Inputs=**  RndMeth=Zero
  tVec2 : Product  Inputs=**  RndMeth=Zero
  v_n : DotProduct  InputSameDT=on  OutDataTypeStr=Inherit: Inherit via internal rule
  v_nVec : Product  RndMeth=Zero
  v_tVec : Sum  Inputs=-+|
  F_n Stick [N N N] : Outport  OutputWhenDisabled=reset  InitialOutput=[0 0 0]
      settings: AttributesFormatString=initial = '%<InitialOutput>'\nwhen disabled = '%<OutputWhenDisabled>'
  F_t Stick [N N N] : Outport  Port=2  OutputWhenDisabled=reset  InitialOutput=[0 0 0]
      settings: AttributesFormatString=when disabled: %<OutputWhenDisabled>\ninitial: %<InitialOutput>
  Sliding! : Outport  Port=3  OutputWhenDisabled=reset  InitialOutput=0
      settings: AttributesFormatString=when disabled: %<OutputWhenDisabled>\ninitial: %<InitialOutput>
  wires:
  Sum/1 -> Positive/1
  Memory/1 -> FixPt Relational Operator/2
  Positive/1 -> FixPt Relational Operator/1, Memory/1
  FixPt Relational Operator/1 -> Sliding!/1
  Abs/1 -> Sum/1
  stiction limit force/1 -> Abs/1
  Positive1/1 -> Check Vertical Friction/2
  Check Vertical Friction/1 -> Vector Norm/1(vec), F_t Stick [N N N]/1
  Normal Ground Reaction Force/1 -> Product1/2, stiction limit force/1, Positive1/1
  Mux2/1 -> Normal Ground Reaction Force/1
  Gain1/1 -> Mux2/1
  Gain2/1 -> Mux2/2
  nVecFP [m m m]/1 -> d_n/1, v_n/2, Dpos_n/1, Dpos_nVec/1, v_nVec/2, Product1/1
  d_n/1 -> Gain1/1
  vel [m/s m/s m/s]/1 -> v_tVec/2, v_n/1
  v_n/1 -> v_nVec/1, Gain2/1
  v_nVec/1 -> v_tVec/1
  v_tVec/1 -> Gain5/1
  Product1/1 -> F_n Stick [N N N]/1
  pos [m]/1 -> Sum2/1, Sum1/2
  posFP [m]/1 -> Sum2/2
  Sum2/1 -> Dpos_n/2, Dpos_tVec/1  "Dpos"
  Dpos_n/1 -> Dpos_nVec/2
  Dpos_nVec/1 -> Dpos_tVec/2
  Dpos_tVec/1 -> Gain3/1
  Gain3/1 -> Sign/1, tVec2/2
  Sign/1 -> tVec1/2
  tVec1/1 -> sum/2
  Constant/1 -> sum/1
  sum/1 -> tVec2/1
  tVec2/1 -> Gain/1
  Gain/1 -> Check Vertical Friction/1
  Vector Norm/1(norm) -> Sum/2
  RefPtFP [m m m]/1 -> Sum1/1
  Sum1/1 -> d_n/2
  Gain5/1 -> tVec1/1

== system nms_3Dmodel_nonlin/Body Mechanics Layer/LLHeel Cnt/3D Contact/Friction Switch ==
  note: Static/Kinetic Friction Switch
  Slide! : Inport
  Stick! : Inport  Port=2
  Memory : Memory
  S-R Flip-Flop : simulink_extras/Flip Flops/S-R Flip-Flop  initial_condition=0
  Terminator : Terminator
  Stiction : Outport
  wires:
  S-R Flip-Flop/1 -> Memory/1
  S-R Flip-Flop/2 -> Terminator/1
  Stick!/1 -> S-R Flip-Flop/1
  Slide!/1 -> S-R Flip-Flop/2
  Memory/1 -> Stiction/1

== system nms_3Dmodel_nonlin/Body Mechanics Layer/LLHeel Cnt/3D Contact/Kinetic Friction Model ==
  note: Kinetic Friction Model
  note: Footpoint Determiner
  note: Sliding Limit Detector
  note: Normal Ground Friction
  note: Tangential Ground Friction
  vel [m/s m/s m/s] : Inport
  pos [m m m] : Inport  Port=2
  RefPt [m m m] : Inport  Port=3
  nVec [m m m] : Inport  Port=4
  Enable : EnablePort  StatesWhenEnabling=reset  ZeroCross=off
  Constant : Constant  Value=vLimit
  Constant1 : Constant  Value=[0 0 0 1]'
  Demux : Demux  Outputs=[3 1]
  FixPt Relational Operator : RelationalOperator  Operator=>  OutDataTypeStr=boolean  ZeroCross=off  RndMeth=Nearest
  Gain3 : Gain  Gain=k_gn
  Gain4 : Gain  Gain=1/v_gn_max
  Memory : Memory
  Mux1 : Mux  Inputs=2
  Mux2 : Mux  Inputs=2
  Negative : simulink/Logic and Bit Operations/Compare To Zero  relop=<  OutDataTypeStr=boolean
  Normal Axis Ground Force : Fcn  Expr="u(1)  *  (1-u(2)) * (u(2)<1)"
  Product : Product  RndMeth=Zero
  Product1 : Product  RndMeth=Zero
  Sum : Sum  Inputs=|+-
  Switch : Switch  Criteria=u2 > Threshold  Threshold=0.9*vLimit
      settings: AttributesFormatString=>%<Threshold>?
  Vector Norm : Subsystem
  d_n : DotProduct  InputSameDT=on  OutDataTypeStr=Inherit: Inherit via internal rule
  qnVec : Sum  Inputs=-+
  reverse direction : Gain  Gain=-1
  sliding friction coefficient : Gain  Gain=mu_slide
  tVec : Product  Inputs=*/  RndMeth=Zero
  v_n : DotProduct  InputSameDT=on  OutDataTypeStr=Inherit: Inherit via internal rule
  v_nVec : Product  RndMeth=Zero
  v_tVec : Sum  Inputs=-+|
  RefPtFP [m m m] : Outport  InitialOutput=[0 0 0]
      settings: AttributesFormatString=initial = '%<InitialOutput>'\nwhen disabled = '%<OutputWhenDisabled>'
  posFP [m m m] : Outport  Port=2  InitialOutput=[0 0 0]
      settings: AttributesFormatString=initial = '%<InitialOutput>'\nwhen disabled = '%<OutputWhenDisabled>'
  nVec FP [m m m] : Outport  Port=3  InitialOutput=0
      settings: AttributesFormatString=initial = '%<InitialOutput>'\nwhen disabled = '%<OutputWhenDisabled>'
  Stiction! : Outport  Port=4  OutputWhenDisabled=reset  InitialOutput=0
      settings: AttributesFormatString=initial = '%<InitialOutput>'\nwhen disabled = '%<OutputWhenDisabled>'
  F_t Slide [N N N] : Outport  Port=5  OutputWhenDisabled=reset  InitialOutput=[0 0 0]
      settings: AttributesFormatString=initial = '%<InitialOutput>'\nwhen disabled = '%<OutputWhenDisabled>'
  F_n Slide [N N N] : Outport  Port=6  OutputWhenDisabled=reset  InitialOutput=[0 0 0]
      settings: AttributesFormatString=initial = '%<InitialOutput>'\nwhen disabled = '%<OutputWhenDisabled>'
  wires:
  Normal Axis Ground Force/1 -> sliding friction coefficient/1, Product1/2
  Product/1 -> F_t Slide [N N N]/1
  FixPt Relational Operator/1 -> Stiction!/1
  Memory/1 -> FixPt Relational Operator/2
  Negative/1 -> FixPt Relational Operator/1, Memory/1
  Vector Norm/1(norm) -> Sum/1, Switch/2, Mux2/2
  Sum/1 -> Negative/1
  Constant/1 -> Sum/2
  Mux1/1 -> Normal Axis Ground Force/1
  Gain3/1 -> Mux1/1
  Gain4/1 -> Mux1/2
  nVec [m m m]/1 -> v_n/1, v_nVec/2, d_n/2, Product1/1, nVec FP [m m m]/1
  d_n/1 -> Gain3/1
  vel [m/s m/s m/s]/1 -> v_n/2, v_tVec/2
  v_n/1 -> Gain4/1, v_nVec/1
  v_nVec/1 -> v_tVec/1
  v_tVec/1 -> Vector Norm/1(vec), Mux2/1
  sliding friction coefficient/1 -> Product/1
  reverse direction/1 -> Product/2
  Product1/1 -> F_n Slide [N N N]/1
  tVec/1 -> reverse direction/1
  Constant1/1 -> Switch/3
  Mux2/1 -> Switch/1
  Switch/1 -> Demux/1
  Demux/2 -> tVec/2
  Demux/1 -> tVec/1
  pos [m m m]/1 -> posFP [m m m]/1, qnVec/1
  qnVec/1 -> d_n/1
  RefPt [m m m]/1 -> qnVec/2, RefPtFP [m m m]/1

== system nms_3Dmodel_nonlin/Body Mechanics Layer/LLHeel Cnt/3D Contact/Static Friction Model ==
  note: Stiction Limit Detector
  note: Static Friction Model
  note: Zero multiplication prevents
      | horizontal friction model from
      | oscillating between static and kinetic
      | friction when the vertical force is zero but
      | the ground level is not yet reached
      | in the upward motion
  note: (distance to
      | surface)
  note: Tangential Ground Reaction Force
  pos [m] : Inport
  vel [m/s m/s m/s] : Inport  Port=2
  RefPtFP [m m m] : Inport  Port=3
  posFP [m] : Inport  Port=4
  nVecFP [m m m] : Inport  Port=5
  Enable : EnablePort  StatesWhenEnabling=reset  ZeroCross=off
  Abs : Abs
  Check Vertical Friction : Product  RndMeth=Zero
  Constant : Constant
  Dpos_n : DotProduct  InputSameDT=on  OutDataTypeStr=Inherit: Inherit via internal rule
  Dpos_nVec : Product  RndMeth=Zero
  Dpos_tVec : Sum  Inputs=|+-
  FixPt Relational Operator : RelationalOperator  Operator=>  OutDataTypeStr=boolean  ZeroCross=off  RndMeth=Nearest
  Gain : Gain  Gain=-1
  Gain1 : Gain  Gain=k_gn
  Gain2 : Gain  Gain=1/v_gn_max
  Gain3 : Gain  Gain=k_gt
  Gain5 : Gain  Gain=1/v_gt_max
  Memory : Memory
  Mux2 : Mux  Inputs=2
  Normal Ground Reaction Force : Fcn  Expr="u(1)  *  (1-u(2)) * (u(2)<1)"
  Positive : simulink/Logic and Bit Operations/Compare To Zero  relop=>  OutDataTypeStr=boolean
  Positive1 : simulink/Logic and Bit Operations/Compare To Zero  relop=>  OutDataTypeStr=boolean
  Product1 : Product  RndMeth=Zero
  Sign : Signum  ZeroCross=off
  Sum : Sum  Inputs=-+
  Sum1 : Sum  Inputs=|+-
  Sum2 : Sum  Inputs=|+-
  Vector Norm : Subsystem
  d_n : DotProduct  InputSameDT=on  OutDataTypeStr=Inherit: Inherit via internal rule
  stiction limit force : Gain  Gain=mu_stick
  sum : Sum  Inputs=++|
  tVec1 : Product  Inputs=**  RndMeth=Zero
  tVec2 : Product  Inputs=**  RndMeth=Zero
  v_n : DotProduct  InputSameDT=on  OutDataTypeStr=Inherit: Inherit via internal rule
  v_nVec : Product  RndMeth=Zero
  v_tVec : Sum  Inputs=-+|
  F_n Stick [N N N] : Outport  OutputWhenDisabled=reset  InitialOutput=[0 0 0]
      settings: AttributesFormatString=initial = '%<InitialOutput>'\nwhen disabled = '%<OutputWhenDisabled>'
  F_t Stick [N N N] : Outport  Port=2  OutputWhenDisabled=reset  InitialOutput=[0 0 0]
      settings: AttributesFormatString=when disabled: %<OutputWhenDisabled>\ninitial: %<InitialOutput>
  Sliding! : Outport  Port=3  OutputWhenDisabled=reset  InitialOutput=0
      settings: AttributesFormatString=when disabled: %<OutputWhenDisabled>\ninitial: %<InitialOutput>
  wires:
  Sum/1 -> Positive/1
  Memory/1 -> FixPt Relational Operator/2
  Positive/1 -> FixPt Relational Operator/1, Memory/1
  FixPt Relational Operator/1 -> Sliding!/1
  Abs/1 -> Sum/1
  stiction limit force/1 -> Abs/1
  Positive1/1 -> Check Vertical Friction/2
  Check Vertical Friction/1 -> Vector Norm/1(vec), F_t Stick [N N N]/1
  Normal Ground Reaction Force/1 -> Product1/2, stiction limit force/1, Positive1/1
  Mux2/1 -> Normal Ground Reaction Force/1
  Gain1/1 -> Mux2/1
  Gain2/1 -> Mux2/2
  nVecFP [m m m]/1 -> d_n/1, v_n/2, Dpos_n/1, Dpos_nVec/1, v_nVec/2, Product1/1
  d_n/1 -> Gain1/1
  vel [m/s m/s m/s]/1 -> v_tVec/2, v_n/1
  v_n/1 -> v_nVec/1, Gain2/1
  v_nVec/1 -> v_tVec/1
  v_tVec/1 -> Gain5/1
  Product1/1 -> F_n Stick [N N N]/1
  pos [m]/1 -> Sum2/1, Sum1/2
  posFP [m]/1 -> Sum2/2
  Sum2/1 -> Dpos_n/2, Dpos_tVec/1  "Dpos"
  Dpos_n/1 -> Dpos_nVec/2
  Dpos_nVec/1 -> Dpos_tVec/2
  Dpos_tVec/1 -> Gain3/1
  Gain3/1 -> Sign/1, tVec2/2
  Sign/1 -> tVec1/2
  tVec1/1 -> sum/2
  Constant/1 -> sum/1
  sum/1 -> tVec2/1
  tVec2/1 -> Gain/1
  Gain/1 -> Check Vertical Friction/1
  Vector Norm/1(norm) -> Sum/2
  RefPtFP [m m m]/1 -> Sum1/1
  Sum1/1 -> d_n/2
  Gain5/1 -> tVec1/1

== system nms_3Dmodel_nonlin/Body Mechanics Layer/LMBall Cnt/3D Contact/Friction Switch ==
  note: Static/Kinetic Friction Switch
  Slide! : Inport
  Stick! : Inport  Port=2
  Memory : Memory
  S-R Flip-Flop : simulink_extras/Flip Flops/S-R Flip-Flop  initial_condition=0
  Terminator : Terminator
  Stiction : Outport
  wires:
  S-R Flip-Flop/1 -> Memory/1
  S-R Flip-Flop/2 -> Terminator/1
  Stick!/1 -> S-R Flip-Flop/1
  Slide!/1 -> S-R Flip-Flop/2
  Memory/1 -> Stiction/1
